simulink model "KTH_103002"  (Simulink 4.00)
settings: Solver=FixedStepDiscrete  StartTime=0.0  StopTime=5  RelTol=1e-3
values from neighbouring files (symbols this model uses):
  p2_1050 = [1.65 1.7 1.75 1.8 1.83 1.88 1.92 1.96 2.13 2.35 2.57 2.72 2.85 2.95]    [Comp1050_2.m]
  Pcomp_1050 = [690 790 880 1040 1160 1320 1580 1730 2970 5000 7960 9970 13200 16700]    [Comp1050_2.m]
  Qm_1050 = [2 2.5 3 4.5 5 6.5 8.5 10 20 35 55 65 85 100]    [Comp1050_2.m]
  T2_1050 = [99.2 103.5 107.2 110.7 111.8 112 111.7 100.4 116.5 131.5 136.4 147.4 149.6 155]    [Comp1050_2.m]
undefined symbols (not defined in the file or in its folder): conda, fan_cool, FC, fc_act, fc_blower_rec_H2, fc_blowera, fc_compressor, fc_condc, fc_coolstack, fc_current, fc_eqs, fc_evapcool, pump2, pump_cool, pump_re, radiator, vent
(part 1 of 2)
settings Model: LastModifiedBy=kharalds

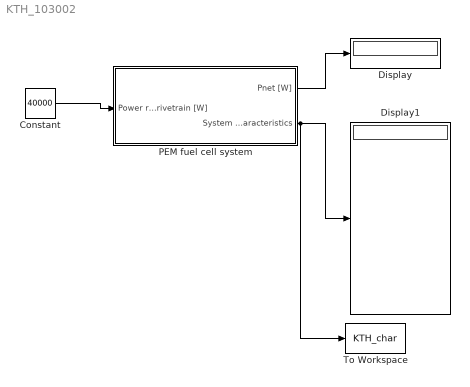
== system KTH_103002 ==
  Constant : Constant  Value=40000
  Display : Display
      settings: Format=short
  Display1 : Display
      settings: Format=short
  PEM fuel cell system : Subsystem
      settings: RTWFcnNameOpts=Auto  RTWFileNameOpts=Auto
  To Workspace : ToWorkspace  VariableName=KTH_char  SampleTime=-1  SaveFormat=Array
  wires:
  PEM fuel cell system/2(System characteristics) -> Display1/1, To Workspace/1
  PEM fuel cell system/1(Pnet [W]) -> Display/1
  Constant/1 -> PEM fuel cell system/1("Power request from drivetrain [W] ")

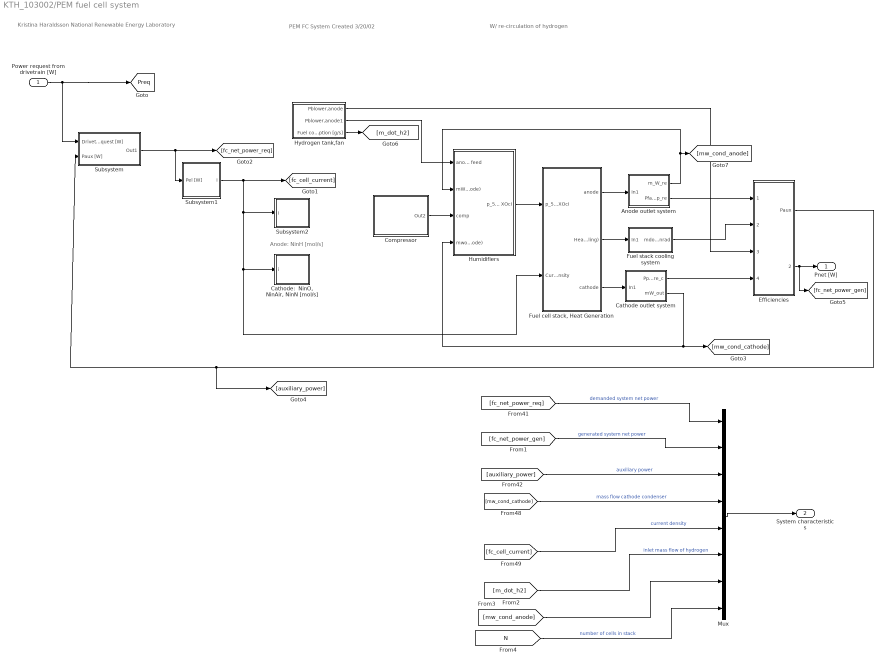
== system KTH_103002/PEM fuel cell system ==
  note: Kristina Haraldsson
      | National Renewable Energy Laboratory
  note: PEM FC System
      | Created  3/20/02
  note: W/ re-circulation of hydrogen
  note: Anode: NinH [mol/s]
  "Power request from drivetrain [W] " : Inport  Port=1  LatchInput=off
  Anode outlet system : Subsystem
      settings: RTWFcnNameOpts=Auto  RTWFileNameOpts=Auto
  Cathode outlet system : Subsystem
      settings: RTWFcnNameOpts=Auto  RTWFileNameOpts=Auto
  "Cathode:  NinO, NinAir, NinN [mol/s]" : Subsystem
      settings: RTWFcnNameOpts=Auto  RTWFileNameOpts=Auto
  "Compressor " : Subsystem
      settings: RTWFcnNameOpts=Auto  RTWFileNameOpts=Auto
  Efficiencies : Subsystem
      settings: RTWFcnNameOpts=Auto  RTWFileNameOpts=Auto
  "Fuel cell stack, Heat Generation" : Subsystem
      settings: RTWFcnNameOpts=Auto  RTWFileNameOpts=Auto
  Fuel stack cooling system : Subsystem
      settings: RTWFcnNameOpts=Auto  RTWFileNameOpts=Auto
  Humidifiers : Subsystem
      settings: RTWFcnNameOpts=Auto  RTWFileNameOpts=Auto
  Hydrogen tank,fan : Subsystem
      settings: RTWFcnNameOpts=Auto  RTWFileNameOpts=Auto
  Mux : Mux  Inputs=8
  Subsystem : Subsystem
      settings: RTWFcnNameOpts=Auto  RTWFileNameOpts=Auto
  Subsystem1 : Subsystem
      settings: RTWFcnNameOpts=Auto  RTWFileNameOpts=Auto
  Subsystem2 : Subsystem
      settings: RTWFcnNameOpts=Auto  RTWFileNameOpts=Auto
  Pnet [W] : Outport  Port=1
  System characteristics : Outport  Port=2
  tag scope: Preq=global
  wires:
  Humidifiers/1("p_56 anode feed p_57 cathode feed Psat Psatah Psatch XWaI,  XWcI  XOcI ") -> "Fuel cell stack, Heat Generation"/1("p_56, NinH, p_57, NinAir, Psat,Psatah,PsatchXWaI, XWcI, XOcI")
  "Compressor "/1(Out2) -> Humidifiers/3(comp)
  "Fuel cell stack, Heat Generation"/1(anode) -> Anode outlet system/1(In1)
  "Fuel cell stack, Heat Generation"/2(Heat_fc (fuel cell stack cooling)) -> Fuel stack cooling system/1(In1)
  Fuel stack cooling system/1(mdotW P_pump A Heat Qcool P_fanrad) -> Efficiencies/2(P_pump,cool P_fanrad)
  Anode outlet system/2(Pfan Ppump_re) -> Efficiencies/1("P_fan_,re, P_pump_re_a")
  Anode outlet system/1(m_W_re) -> Humidifiers/2(mW_out(anode)), [mw_cond_anode]
  "Fuel cell stack, Heat Generation"/3(cathode) -> Cathode outlet system/1(In1)
  Cathode outlet system/1(Ppump_re_c) -> Efficiencies/4(P_pump_re_c)
  Cathode outlet system/2(mW_out) -> Humidifiers/4(mwout(cathode)), [mw_cond_cathode]
  Hydrogen tank,fan/1(Pblower,anode) -> Efficiencies/3(P_fan,anode)
  Efficiencies/1(Paux) -> Subsystem/2(Paux [W]), [auxiliary_power]
  Subsystem/1(Out1) -> Subsystem1/1(Pel [W]), [fc_net_power_req]
  "Power request from drivetrain [W] "/1 -> Subsystem/1(Drivetrain Power Request [W]), [Preq]
  Subsystem1/1(i) -> Subsystem2/1(i), "Cathode:  NinO, NinAir, NinN [mol/s]"/1(i), "Fuel cell stack, Heat Generation"/2(Current density), [fc_cell_current]
  Efficiencies/2(Pnet [W]) -> Pnet [W]/1, [fc_net_power_gen]
  Hydrogen tank,fan/3(Fuel consumption [g/s]) -> [m_dot_h2]
  Hydrogen tank,fan/2(Pblower,anode1) -> Humidifiers/1(anode feed)
  [fc_net_power_req] -> Mux/1  "demanded system net power"
  [auxiliary_power] -> Mux/3  "auxiliary power"
  [mw_cond_cathode] -> Mux/4  "mass flow cathode condenser"
  [fc_cell_current] -> Mux/5  "current density"
  [fc_net_power_gen] -> Mux/2  "generated system net power"
  Mux/1 -> System characteristics/1
  [m_dot_h2] -> Mux/6  "inlet mass flow of hydrogen"
  [mw_cond_anode] -> Mux/7
  [N] -> Mux/8  "number of cells in stack"

== system KTH_103002/PEM fuel cell system/Anode outlet system ==
  note: FCSystem_H2/Anode outlet system
  In1 : Inport  Port=1  LatchInput=off
  Anode condenser : Subsystem
      settings: RTWFcnNameOpts=Auto  RTWFileNameOpts=Auto
  Mux : Mux  Inputs=2
  Mux1 : Mux  Inputs=2
  "Re-circulation: Blower_rec, pump" : Subsystem
      settings: RTWFcnNameOpts=Auto  RTWFileNameOpts=Auto
  Vent/Purge : Subsystem
      settings: RTWFcnNameOpts=Auto  RTWFileNameOpts=Auto
  m_W_re : Outport  Port=1
  Pfan Ppump_re : Outport  Port=2
  tag scope: NoutH=global
  wires:
  In1/1 -> Anode condenser/1(In1)
  Anode condenser/1(Out1) -> Vent/Purge/1(In1)
  Vent/Purge/1(Out1) -> "Re-circulation: Blower_rec, pump"/1(In1)
  "Re-circulation: Blower_rec, pump"/3(p_70) -> Mux/2
  "Re-circulation: Blower_rec, pump"/4(Pfan) -> Mux1/1
  "Re-circulation: Blower_rec, pump"/5(Ppump_re) -> Mux1/2
  Mux1/1 -> Pfan Ppump_re/1
  "Re-circulation: Blower_rec, pump"/1(m_W_re) -> m_W_re/1
  "Re-circulation: Blower_rec, pump"/2(NoutH_re) -> Mux/1
  Mux/1 -> [NoutH]

== system KTH_103002/PEM fuel cell system/Cathode outlet system ==
  note: FCSystem/Cathode outlet system
  In1 : Inport  Port=1  LatchInput=off
  Cathode condenser : Subsystem
      settings: RTWFcnNameOpts=Auto  RTWFileNameOpts=Auto
  Pump (cathode) : Subsystem
      settings: RTWFcnNameOpts=Auto  RTWFileNameOpts=Auto
  Ppump_re_c : Outport  Port=1
  mW_out : Outport  Port=2
  wires:
  In1/1 -> Cathode condenser/1(In1)
  Pump (cathode)/1(Ppump_re_c) -> Ppump_re_c/1
  Cathode condenser/1(mw_out1) -> Pump (cathode)/1(In1)
  Pump (cathode)/2(mW_out) -> mW_out/1

== system KTH_103002/PEM fuel cell system/Cathode:  NinO, NinAir, NinN [mol/s] ==
  note: Total cathode molar flow
  i : Inport  Port=1  LatchInput=off
  Constant : Constant  Value=FC.Lab.Stoich.vO
  Constant1 : Constant  Value=FC.Stack.Cell.Dim.A
  Constant2 : Constant  Value=FC.Stack.N
  Constant3 : Constant  Value=FC.Const.F
  Constant4 : Constant  Value=4
  Constant5 : Constant  Value=FC.Lab.Stoich.XON
  Constant6 : Constant  Value=FC.Lab.Stoich.XON
  Constant7 : Constant  Value=1
  Constant8 : Constant  Value=FC.Const.Mair
  Display{,1..3} (4 alike) : Display
      settings: Format=short
  Product : Product  Inputs=4  Multiplication=Element-wise(.*)  SaturateOnIntegerOverflow=on
  Product1 : Product  Inputs=*/  Multiplication=Element-wise(.*)  SaturateOnIntegerOverflow=on
  Product2 : Product  Inputs=2  Multiplication=Element-wise(.*)  SaturateOnIntegerOverflow=on
  Product3 : Product  Inputs=*/  Multiplication=Element-wise(.*)  SaturateOnIntegerOverflow=on
  Product4 : Product  Inputs=2  Multiplication=Element-wise(.*)  SaturateOnIntegerOverflow=on
  Product5 : Product  Inputs=2  Multiplication=Element-wise(.*)  SaturateOnIntegerOverflow=on
  Sum : Sum  Inputs=|+-  SaturateOnIntegerOverflow=on
  tag scope: NinAir=global, NinN=global, NinO=global
  wires:
  Constant1/1 -> Product/3
  Constant/1 -> Product/2
  i/1 -> Product/1
  Constant2/1 -> Product/4
  Product/1 -> Product1/1
  Constant4/1 -> Product2/2
  Product2/1 -> Product1/2
  Product1/1 -> Product3/1, [NinO], Display/1
  Constant5/1 -> Product3/2
  Product3/1 -> Product4/1, [NinAir], Display1/1, Product5/1
  Constant7/1 -> Sum/1
  Constant6/1 -> Sum/2
  Sum/1 -> Product4/2
  Product4/1 -> [NinN], Display2/1
  Constant3/1 -> Product2/1
  Constant8/1 -> Product5/2
  Product5/1 -> Display3/1

== system KTH_103002/PEM fuel cell system/Compressor  ==
  note: FCSystem_H2/Compressor
  "Initial value, 0.1 mole/s" : Memory  X0=0.1  InheritSampleTime=off
      settings: RTWStateStorageClass=Auto
  M_air [g/mol] : Constant  Value=FC.Const.Mair
  M_air [g/mol]1 : Constant  Value=FC.Lab.P.c
  Mass flow [g/s]  discharge pressure [bar(a)] CompOA1050 (Opcon) : Lookup  InputValues=[Qm_1050]  OutputValues=[p2_1050]
  Mass flow [g/s] Pcomp [W] CompOA1050 (Opcon) : Lookup  InputValues=[Qm_1050]  OutputValues=[Pcomp_1050]
  Mass flow [g/s] discharge temperature [C] CompOA1050 (Opcon)1 : Lookup  InputValues=[Qm_1050]  OutputValues=[T2_1050]
  Mux : Mux  Inputs=5
  P1 : Display
      settings: Format=short
  P2 : Display
      settings: Format=short
  Pcomp1 : Display
      settings: Format=short
  Product : Product  Inputs=2  Multiplication=Element-wise(.*)  SaturateOnIntegerOverflow=on
  Selector : Selector  InputType=Vector  ElementSrc=Internal  Elements=[4]  RowSrc=Internal  Rows=1  ColumnSrc=Internal  Columns=1  InputPortWidth=7
  fc_compressor.m : MATLABFcn  MATLABFcn=fc_compressor(u,FC.Lab.P.amb,FC.Lab.Temp.amb,FC.Const.eta1,FC.Const.etagen,FC.Lab.Stoich.RHo,FC.Lab.P.hum,FC.Lab.Temp.evap,FC.Lab.Temp.cell,FC.Stack.Pel)  OutputDimensions=7  OutputSignalType=auto  Output1D=on
  Out2 : Outport  Port=1
  tag scope: P_comp=global
  wires:
  M_air [g/mol]/1 -> Product/2
  Mux/1 -> fc_compressor.m/1
  Selector/1 -> Pcomp1/1, [P_comp]
  fc_compressor.m/1 -> Out2/1, Selector/1
  Mass flow [g/s]  discharge pressure [bar(a)] CompOA1050 (Opcon)/1 -> Mux/2, P2/1
  Mass flow [g/s] Pcomp [W] CompOA1050 (Opcon)/1 -> Mux/3
  [NinAir] -> "Initial value, 0.1 mole/s"/1
  "Initial value, 0.1 mole/s"/1 -> Mux/1, Product/1
  Product/1 -> Mass flow [g/s]  discharge pressure [bar(a)] CompOA1050 (Opcon)/1, Mass flow [g/s] Pcomp [W] CompOA1050 (Opcon)/1, Mass flow [g/s] discharge temperature [C] CompOA1050 (Opcon)1/1, P1/1
  Mass flow [g/s] discharge temperature [C] CompOA1050 (Opcon)1/1 -> Mux/4
  M_air [g/mol]1/1 -> Mux/5

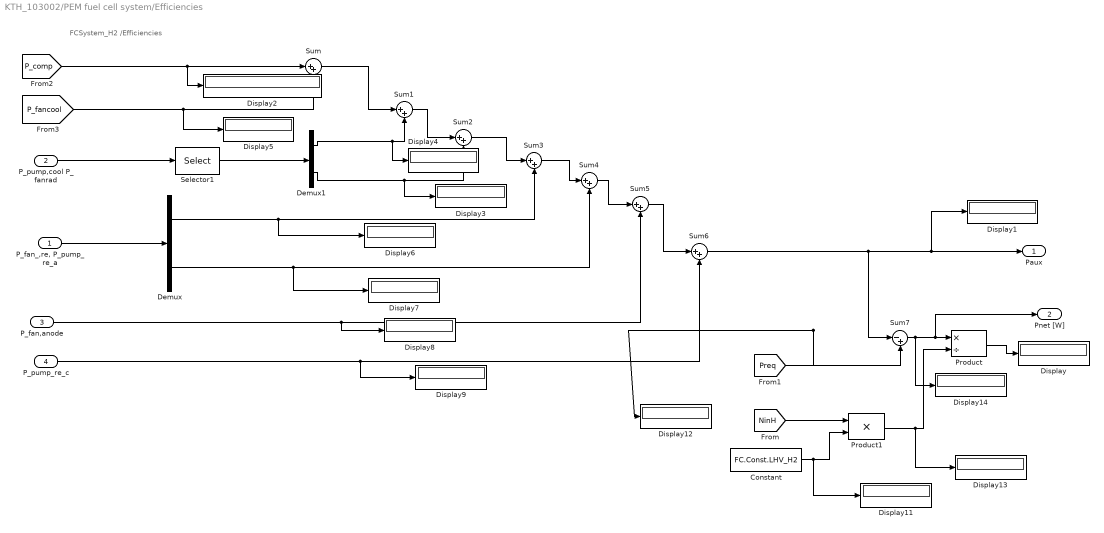
== system KTH_103002/PEM fuel cell system/Efficiencies ==
  note: FCSystem_H2
      | /Efficiencies
  "P_fan_,re, P_pump_re_a" : Inport  Port=1  LatchInput=off
  P_pump,cool P_fanrad : Inport  Port=2  LatchInput=off
  P_fan,anode : Inport  Port=3  LatchInput=off
  P_pump_re_c : Inport  Port=4  LatchInput=off
  Constant : Constant  Value=FC.Const.LHV_H2
  Demux : Demux  Outputs=2  BusSelectionMode=off
  Demux1 : Demux  Outputs=2  BusSelectionMode=off
  Display{,1..9,11..14} (14 alike) : Display
      Display settings: Format=short
      Display1 settings: Format=short
      Display11 settings: Format=short
      Display12 settings: Format=short
      Display13 settings: Format=short
      Display14 settings: Format=short
      Display3 settings: Format=short
      Display4 settings: Format=short
      Display5 settings: Format=short
      Display6 settings: Format=short
      Display7 settings: Format=short
      Display8 settings: Format=short
      Display9 settings: Format=short
  Product : Product  Inputs=*/  Multiplication=Element-wise(.*)  SaturateOnIntegerOverflow=on
  Product1 : Product  Inputs=2  Multiplication=Element-wise(.*)  SaturateOnIntegerOverflow=on
  Selector1 : Selector  InputType=Vector  ElementSrc=Internal  Elements=[2 6]  RowSrc=Internal  Rows=1  ColumnSrc=Internal  Columns=1  InputPortWidth=6
  Sum{,1..6} (7 alike) : Sum  Inputs=|++  SaturateOnIntegerOverflow=on
  Sum7 : Sum  Inputs=|-+  SaturateOnIntegerOverflow=on
  Paux : Outport  Port=1
  Pnet [W] : Outport  Port=2
  wires:
  P_pump,cool P_fanrad/1 -> Selector1/1
  [P_comp] -> Sum/1, Display2/1
  "P_fan_,re, P_pump_re_a"/1 -> Demux/1
  P_pump_re_c/1 -> Sum6/2, Display9/1
  P_fan,anode/1 -> Sum5/2, Display8/1
  Demux/1 -> Sum3/2, Display6/1
  Demux/2 -> Sum4/2, Display7/1
  [P_fancool] -> Sum/2, Display5/1
  Sum/1 -> Sum1/1
  Selector1/1 -> Demux1/1
  Demux1/1 -> Sum1/2, Display4/1
  Sum1/1 -> Sum2/1
  Demux1/2 -> Sum2/2, Display3/1
  Sum2/1 -> Sum3/1
  Sum3/1 -> Sum4/1
  Sum4/1 -> Sum5/1
  Sum5/1 -> Sum6/1
  Sum6/1 -> Sum7/1, Paux/1, Display1/1
  Sum7/1 -> Display14/1, Product/1, Pnet [W]/1
  [Preq] -> Sum7/2, Display12/1
  Constant/1 -> Product1/2, Display11/1
  [NinH] -> Product1/1
  Product1/1 -> Product/2, Display13/1
  Product/1 -> Display/1

== system KTH_103002/PEM fuel cell system/Fuel cell stack, Heat Generation ==
  note: FCSystem_H2
      | /Fuel cell stack, Heat generation
  note: NinWa NinHa NoutWag NoutHa
      | NinWc NinO NinN NoutWcg NWlgen
      | NoutWcl NoutO NoutN Nout_condc Nout_conda
  "p_56, NinH, p_57, NinAir, Psat,Psatah,PsatchXWaI, XWcI, XOcI" : Inport  Port=1  LatchInput=off
  Current density : Inport  Port=2  LatchInput=off
  Constant1 : Constant  Value=FC.Const.F
  Constant3 : Constant  Value=2
  Display{,1..3} (4 alike) : Display
      settings: Format=short
  Heat : Subsystem
      settings: RTWFcnNameOpts=Auto  RTWFileNameOpts=Auto
  J Water produced at cathode : Product  Inputs=/*  Multiplication=Element-wise(.*)  SaturateOnIntegerOverflow=on
  Mux1 : Mux  Inputs=5
  Product2 : Product  Inputs=2  Multiplication=Element-wise(.*)  SaturateOnIntegerOverflow=on
  fc_eqs : MATLABFcn  MATLABFcn=fc_eqs(u, FC.Stack.Cell.Dim.A, FC.Lab.P.a,FC.Lab.P.c,FC.Lab.P.amb,FC.Lab.Stoich.RHo,FC.Const.F,FC.Lab.Temp.cell,FC.Lab.Temp.ah,FC.Lab.Temp.ch,FC.Lab.Temp.amb,FC.Stack.Cell.Memb.Mm,FC.Stack.Cell.Memb.pdry,FC.Stack.Cell.Dim.tm,FC.Lab.Stoich.vO,FC.Lab.Stoich.vH,FC.Const.zw,FC.Stack.Pel,FC.Stack.N)  OutputDimensions=20  OutputSignalType=auto  Output1D=on
  flows : Selector  InputType=Vector  ElementSrc=Internal  Elements=[3 4 5 6 7 8 10 11 12 13 14 19 20]  RowSrc=Internal  Rows=1  ColumnSrc=Internal  Columns=1  InputPortWidth=20
  flows p_60 NoutWcg NoutWlgen NoutWcl NoutO NoutN Nout_condc : Selector  InputType=Vector  ElementSrc=Internal  Elements=[1 10 11 12 13 14 19]  RowSrc=Internal  Rows=1  ColumnSrc=Internal  Columns=1  InputPortWidth=20
  "p_61,NoutWag, NoutHa,NWAout,NoutWal" : Selector  InputType=Vector  ElementSrc=Internal  Elements=[2 5 6 16 17]  RowSrc=Internal  Rows=1  ColumnSrc=Internal  Columns=1  InputPortWidth=20
  anode : Outport  Port=1
  Heat_fc (fuel cell stack cooling) : Outport  Port=2
  cathode : Outport  Port=3
  tag scope: eta_fc=global
  wires:
  "p_56, NinH, p_57, NinAir, Psat,Psatah,PsatchXWaI, XWcI, XOcI"/1 -> Mux1/1
  "p_61,NoutWag, NoutHa,NWAout,NoutWal"/1 -> anode/1, Display/1
  Mux1/1 -> fc_eqs/1
  fc_eqs/1 -> "p_61,NoutWag, NoutHa,NWAout,NoutWal"/1, flows/1, flows p_60 NoutWcg NoutWlgen NoutWcl NoutO NoutN Nout_condc/1
  flows/1 -> Heat/1(In1 NinWa NinHa NoutWag NoutHa NinWc NinO NinN NoutWcg NoutWcl NoutO NoutN Nout_condc Nout_conda)
  Heat/1(Heat_fc) -> Heat_fc (fuel cell stack cooling)/1, Display3/1
  [NinO] -> Mux1/2
  [NinN] -> Mux1/3
  [lambda] -> Mux1/4
  Current density/1 -> Heat/2(Current density [A/cm2]), J Water produced at cathode/2
  Heat/2(eta_fc) -> [eta_fc], Display2/1
  flows p_60 NoutWcg NoutWlgen NoutWcl NoutO NoutN Nout_condc/1 -> cathode/1, Display1/1
  Constant1/1 -> Product2/1
  Constant3/1 -> Product2/2
  Product2/1 -> J Water produced at cathode/1
  J Water produced at cathode/1 -> Mux1/5

== system KTH_103002/PEM fuel cell system/Fuel stack cooling system ==
  note: FCSystem_H2
      | /Fuel stack cooling system
  note: Cooling medium: air
  note: Cooling medium: water
  In1 : Inport  Port=1  LatchInput=off
  Display : Display
      settings: Format=short
  Display1 : Display
      settings: Format=short
  Pump_cool : Subsystem
      settings: RTWFcnNameOpts=Auto  RTWFileNameOpts=Auto
  Radiator : Subsystem
      settings: RTWFcnNameOpts=Auto  RTWFileNameOpts=Auto
  fan_cool : Subsystem
      settings: RTWFcnNameOpts=Auto  RTWFileNameOpts=Auto
  fuel stack cooling mass flows : Subsystem
      settings: RTWFcnNameOpts=Auto  RTWFileNameOpts=Auto
  mdotW P_pump A Heat Qcool P_fanrad : Outport  Port=1
  tag scope: P_fancool=global
  wires:
  In1/1 -> fuel stack cooling mass flows/1(In1)
  fuel stack cooling mass flows/1(Cooling water flow [kg/s] Cooling air flow [kg/s]) -> Pump_cool/1(In1), fan_cool/1(m_A,T1,Q,etafc)
  fan_cool/1(P_fancool) -> Display/1, [P_fancool]
  Pump_cool/1(Out1) -> Radiator/1(In1)
  Radiator/1(Out2) -> mdotW P_pump A Heat Qcool P_fanrad/1, Display1/1

== system KTH_103002/PEM fuel cell system/Humidifiers ==
  note: FCSystem_H2/Humidifiers
  anode feed : Inport  Port=1  LatchInput=off
  mW_out(anode) : Inport  Port=2  LatchInput=off
  comp : Inport  Port=3  LatchInput=off
  mwout(cathode) : Inport  Port=4  LatchInput=off
  Constant : Constant  Value=FC.Lab.P.c
  Constant1 : Constant  Value=FC.Lab.P.a
  Evapcooler : Subsystem
      settings: RTWFcnNameOpts=Auto  RTWFileNameOpts=Auto
  Memory : Memory  X0=[0.00058799]  InheritSampleTime=off
      settings: RTWStateStorageClass=Auto
  Memory (former value  1.280458) : Memory  X0=0.04  InheritSampleTime=off
      settings: RTWStateStorageClass=Auto
  Mux : Mux  Inputs=6
  Selector : Selector  InputType=Vector  ElementSrc=Internal  Elements=[1 2 3 4 5 6 7 8 9 10 ]  RowSrc=Internal  Rows=1  ColumnSrc=Internal  Columns=1  InputPortWidth=25
  "p_56 anode feed p_57 cathode feed Psat Psatah Psatch XWaI,  XWcI  XOcI " : Outport  Port=1
  wires:
  anode feed/1 -> Evapcooler/1(anode feed Thyd p NinHa Pfan)
  Selector/1 -> "p_56 anode feed p_57 cathode feed Psat Psatah Psatch XWaI,  XWcI  XOcI "/1
  mW_out(anode)/1 -> Memory/1
  Memory/1 -> Evapcooler/2(mW_out(anode))
  mwout(cathode)/1 -> Memory (former value  1.280458)/1
  Evapcooler/1(Out1) -> Selector/1
  [psat_air] -> Mux/1
  [psatah] -> Mux/2
  [psatch] -> Mux/3
  [XWaI] -> Mux/4
  [XWcI] -> Mux/5
  [XOcI] -> Mux/6
  Mux/1 -> Evapcooler/7("Psat,Psatah, PsatchXWaI,  XWcI, XOcI")
  Memory (former value  1.280458)/1 -> Evapcooler/3(mW_out(cathode))
  Constant/1 -> Evapcooler/4(Pc)
  Constant1/1 -> Evapcooler/5(Pa)
  comp/1 -> Evapcooler/6(comp)

== system KTH_103002/PEM fuel cell system/Hydrogen tank,fan ==
  note: FCSystem_H2/Hydrogen tank, fan
  note: Fuel consumption
      | [mol/s]
  Constant : Constant  Value=FC.Const.MH
  Display : Display
      settings: Format=short
  Display1 : Display
      settings: Format=short
  Display2 : Display
      settings: Format=short
  Fcn : Fcn  Expr=u(4)
  Mux : Mux  Inputs=2
  NinH (initial fuel flow) [mol/s]  NinH (fuel cons.) [mol.s] : Selector  InputType=Vector  ElementSrc=Internal  Elements=[2]  RowSrc=Internal  Rows=1  ColumnSrc=Internal  Columns=1  InputPortWidth=2
  Product : Product  Inputs=2  Multiplication=Element-wise(.*)  SaturateOnIntegerOverflow=on
  Selector : Selector  InputType=Vector  ElementSrc=Internal  Elements=[1]  RowSrc=Internal  Rows=1  ColumnSrc=Internal  Columns=1  InputPortWidth=2
  Sum : Sum  Inputs=|+-  SaturateOnIntegerOverflow=on
  blowera.m : MATLABFcn  MATLABFcn=fc_blowera(u,FC.Const.etablow,FC.Stack.dpipe,FC.Stack.Lpipe,FC.Const.g,FC.Lab.P.blowa,FC.Lab.P.an,FC.Lab.P.a,FC.Lab.P.hum,FC.Lab.Temp.cell)  OutputDimensions=4  OutputSignalType=auto  Output1D=on
  Pblower,anode : Outport  Port=1
  Pblower,anode1 : Outport  Port=2
  Fuel consumption [g/s] : Outport  Port=3
  wires:
  blowera.m/1 -> Fcn/1, Pblower,anode1/1
  Fcn/1 -> Pblower,anode/1, Display2/1
  Mux/1 -> NinH (initial fuel flow) [mol/s]  NinH (fuel cons.) [mol.s]/1
  [NinH] -> Sum/1, blowera.m/1, Mux/1
  [NoutH] -> Selector/1
  Constant/1 -> Product/2
  NinH (initial fuel flow) [mol/s]  NinH (fuel cons.) [mol.s]/1 -> Product/1
  Product/1 -> Fuel consumption [g/s]/1
  Selector/1 -> Sum/2, Display/1
  Sum/1 -> Mux/2, Display1/1

== system KTH_103002/PEM fuel cell system/Subsystem ==
  note: Power Request
  Drivetrain Power Request [W] : Inport  Port=1  LatchInput=off
  Paux [W] : Inport  Port=2  LatchInput=off
  Display : Display
      settings: Format=short
  Display1 : Display
      settings: Format=short
  Display2 : Display
      settings: Format=short
  "Inverse of efficiency of DC/DC " : Constant  Orientation=up  Value=1/FC.Const.eta_DCDC
  Memory : Memory  X0=5000  InheritSampleTime=off
      settings: RTWStateStorageClass=Auto
  Preq=(Pel+Paux)/eta_DCDC : Product  Inputs=2  Multiplication=Element-wise(.*)  SaturateOnIntegerOverflow=on
  Sum1 : Sum  Inputs=|++  SaturateOnIntegerOverflow=on
  Out1 : Outport  Port=1
  wires:
  Drivetrain Power Request [W]/1 -> Display2/1, Sum1/1
  Sum1/1 -> Preq=(Pel+Paux)/eta_DCDC/1, Display/1
  "Inverse of efficiency of DC/DC "/1 -> Preq=(Pel+Paux)/eta_DCDC/2
  Preq=(Pel+Paux)/eta_DCDC/1 -> Display1/1, Out1/1
  Paux [W]/1 -> Memory/1
  Memory/1 -> Sum1/2

== system KTH_103002/PEM fuel cell system/Subsystem1 ==
  Pel [W] : Inport  Port=1  LatchInput=off
  Anode init : Subsystem
      settings: RTWFcnNameOpts=Auto  RTWFileNameOpts=Auto
  Cathode Overpotential : Subsystem
      settings: RTWFcnNameOpts=Auto  RTWFileNameOpts=Auto
  Cathode oxygen molar fraction : Subsystem
      settings: RTWFcnNameOpts=Auto  RTWFileNameOpts=Auto
  Cathode water molar fraction : Subsystem
      settings: RTWFcnNameOpts=Auto  RTWFileNameOpts=Auto
  Constant : Constant  Value=FC.Stack.N
  Demux : Demux  Outputs=3  BusSelectionMode=off
  Display{1..4} (4 alike) : Display
      settings: Format=short
  Membrane conductivity : Subsystem
      settings: RTWFcnNameOpts=Auto  RTWFileNameOpts=Auto
  Membrane resistance : Subsystem
      settings: RTWFcnNameOpts=Auto  RTWFileNameOpts=Auto
  Mux : Mux  Inputs=4
  Saturation pressure  cathode humidifier : Subsystem
      settings: RTWFcnNameOpts=Auto  RTWFileNameOpts=Auto
  fc_current : MATLABFcn  MATLABFcn=fc_current(u,FC.Lab.P.c,FC.Lab.P.a,FC.Stack.Cell.Dim.tm,FC.Const.F,FC.Const.jo,FC.Const.Voc,FC.Const.R2,FC.Stack.Cell.Dim.A,FC.Lab.Temp.cell,FC.Lab.Temp.ah,FC.Lab.Temp.ch)  OutputDimensions=3  OutputSignalType=auto  Output1D=on
  i : Outport  Port=1
  tag scope: Ecell=global, N=global, Po=global, Rm=global
  wires:
  Membrane conductivity/1(Sigma) -> Membrane resistance/1(sigma)
  Anode init/1(lambda) -> Membrane conductivity/1(lambda)
  Membrane resistance/1(Rm [ohm/cm2]) -> [Rm], Mux/1
  Saturation pressure  cathode humidifier/1(psatch) -> Cathode water molar fraction/1(psatch [bar])
  Cathode water molar fraction/1(XWcI [-]) -> Cathode Overpotential/2(XWcI), Cathode oxygen molar fraction/1(XWcI [-]1)
  Cathode oxygen molar fraction/1(XOcI [-]) -> Cathode Overpotential/1(XOcI)
  Cathode Overpotential/1(Po) -> [Po], Mux/2
  Mux/1 -> fc_current/1
  Pel [W]/1 -> Mux/3
  fc_current/1 -> Demux/1
  Demux/2 -> [Ecell], Display1/1
  Demux/1 -> i/1, Display4/1
  Demux/3 -> [N], Display2/1
  Constant/1 -> Mux/4, Display3/1

== system KTH_103002/PEM fuel cell system/Subsystem2 ==
  note: Total anode molar flow
  i : Inport  Port=1  LatchInput=off
  Constant : Constant  Value=FC.Lab.Stoich.vH
  Constant1 : Constant  Value=FC.Stack.Cell.Dim.A
  Constant2 : Constant  Value=FC.Stack.N
  Constant3 : Constant  Value=FC.Const.F
  Constant4 : Constant  Value=2
  Constant5 : Constant  Value=FC.Const.MH
  Display : Display
      settings: Format=short
  Display1 : Display
      settings: Format=short
  Product : Product  Inputs=4  Multiplication=Element-wise(.*)  SaturateOnIntegerOverflow=on
  Product1 : Product  Inputs=*/  Multiplication=Element-wise(.*)  SaturateOnIntegerOverflow=on
  Product2 : Product  Inputs=2  Multiplication=Element-wise(.*)  SaturateOnIntegerOverflow=on
  Product3 : Product  Inputs=2  Multiplication=Element-wise(.*)  SaturateOnIntegerOverflow=on
  tag scope: NinH=global
  wires:
  Constant1/1 -> Product/3
  Constant/1 -> Product/2
  i/1 -> Product/1
  Constant2/1 -> Product/4
  Product/1 -> Product1/1
  Constant3/1 -> Product2/1
  Constant4/1 -> Product2/2
  Product2/1 -> Product1/2
  Product1/1 -> [NinH], Display/1, Product3/1
  Constant5/1 -> Product3/2
  Product3/1 -> Display1/1

== system KTH_103002/PEM fuel cell system/Anode outlet system/Anode condenser ==
  note: FCSystem_H2/Anode outlet system/Anode condenser
  In1 : Inport  Port=1  LatchInput=off
  conda : MATLABFcn  MATLABFcn=conda(u,FC.Const.ex,FC.Lab.Temp.amb,FC.Lab.Temp.cond,FC.Lab.Temp.cell)  OutputDimensions=6  OutputSignalType=auto  Output1D=on
  Out1 : Outport  Port=1
  wires:
  In1/1 -> conda/1
  conda/1 -> Out1/1

== system KTH_103002/PEM fuel cell system/Anode outlet system/Re-circulation: Blower_rec, pump ==
  note: FCSystem_H2/Anode outlet system/Blower, pump
  In1 : Inport  Port=1  LatchInput=off
  Demux : Demux  Outputs=2  BusSelectionMode=off
  Demux1 : Demux  Outputs=3  BusSelectionMode=off
  Memory : Memory  X0=0.06848  InheritSampleTime=off
      settings: RTWStateStorageClass=Auto
  Memory1 : Memory  X0=2.59  InheritSampleTime=off
      settings: RTWStateStorageClass=Auto
  Selector1 : Selector  InputType=Vector  ElementSrc=Internal  Elements=[2 3 4]  RowSrc=Internal  Rows=1  ColumnSrc=Internal  Columns=1  InputPortWidth=5
  Selector2 : Selector  InputType=Vector  ElementSrc=Internal  Elements=[1 2]  RowSrc=Internal  Rows=1  ColumnSrc=Internal  Columns=1  InputPortWidth=5
  fc_blower_rec_H2 re-circulation of hydrogen : MATLABFcn  MATLABFcn=fc_blower_rec_H2(u,FC.Const.etablow,FC.Lab.Temp.cell,FC.Stack.dpipe,FC.Stack.Lpipe,FC.Lab.P.blowr,FC.Const.g,FC.Const.MH)  OutputDimensions=5  OutputSignalType=auto  Output1D=on
  pump_re (re-circulation of water from the anode) : MATLABFcn  MATLABFcn=pump_re(u,FC.Lab.Temp.cond,FC.Const.g,FC.Stack.dpipe,FC.Stack.Lpipe,FC.Const.etapump)  OutputDimensions=5  OutputSignalType=auto  Output1D=on
  m_W_re : Outport  Port=1
  NoutH_re : Outport  Port=2
  p_70 : Outport  Port=3
  Pfan : Outport  Port=4
  Ppump_re : Outport  Port=5
  wires:
  In1/1 -> pump_re (re-circulation of water from the anode)/1, fc_blower_rec_H2 re-circulation of hydrogen/1
  pump_re (re-circulation of water from the anode)/1 -> Selector2/1
  Selector2/1 -> Demux/1
  Demux/1 -> Ppump_re/1
  Demux/2 -> m_W_re/1
  Selector1/1 -> Demux1/1
  Demux1/2 -> Memory1/1
  fc_blower_rec_H2 re-circulation of hydrogen/1 -> Selector1/1
  Demux1/1 -> Memory/1
  Memory/1 -> NoutH_re/1
  Memory1/1 -> p_70/1
  Demux1/3 -> Pfan/1

== system KTH_103002/PEM fuel cell system/Anode outlet system/Vent/Purge ==
  note: FCSystem_H2/Anode outlet system/Purge
  In1 : Inport  Port=1  LatchInput=off
  vent : MATLABFcn  MATLABFcn=vent(u,FC.Const.ex)  OutputDimensions=10  OutputSignalType=auto  Output1D=on
  Out1 : Outport  Port=1
  wires:
  In1/1 -> vent/1
  vent/1 -> Out1/1

== system KTH_103002/PEM fuel cell system/Cathode outlet system/Cathode condenser ==
  note: FCSystem/Cathode outlet system/Cathode condenser
  In1 : Inport  Port=1  LatchInput=off
  Mux : Mux  Inputs=2
  Saturation temperature : Subsystem
      settings: RTWFcnNameOpts=Auto  RTWFileNameOpts=Auto
  Selector : Selector  InputType=Vector  ElementSrc=Internal  Elements=[1]  RowSrc=Internal  Rows=1  ColumnSrc=Internal  Columns=1  InputPortWidth=7
  To Workspace : ToWorkspace  VariableName=condc  SampleTime=-1  SaveFormat=Array
  fc_condc : MATLABFcn  MATLABFcn=fc_condc(u,FC.Lab.Temp.amb,FC.Lab.Temp.cond,FC.Lab.Temp.ch,FC.Lab.Temp.cell)  OutputDimensions=7  OutputSignalType=auto  Output1D=on
  mw_out : Selector  InputType=Vector  ElementSrc=Internal  Elements=[4]  RowSrc=Internal  Rows=1  ColumnSrc=Internal  Columns=1  InputPortWidth=7
  mw_out1 : Outport  Port=1
  wires:
  In1/1 -> Mux/1, Selector/1
  fc_condc/1 -> mw_out/1, To Workspace/1
  mw_out/1 -> mw_out1/1
  Mux/1 -> fc_condc/1
  Saturation temperature/1(Temp [K]) -> Mux/2
  Selector/1 -> Saturation temperature/1(pressure [bar])

== system KTH_103002/PEM fuel cell system/Cathode outlet system/Pump (cathode) ==
  note: FCSystem/Cathode outlet system/Pump (cathode)
  note: mw_out
      | condensed water from
      |  the cathode
  In1 : Inport  Port=1  LatchInput=off
  Selector : Selector  InputType=Vector  ElementSrc=Internal  Elements=[2]  RowSrc=Internal  Rows=1  ColumnSrc=Internal  Columns=1  InputPortWidth=2
  Selector1 : Selector  InputType=Vector  ElementSrc=Internal  Elements=[1]  RowSrc=Internal  Rows=1  ColumnSrc=Internal  Columns=1  InputPortWidth=2
  To Workspace : ToWorkspace  VariableName=pump_re_c  SampleTime=-1  SaveFormat=Array
  pump2 (re-circulation of water from the cathode) : MATLABFcn  MATLABFcn=pump2(u,FC.Lab.Temp.cond,FC.Const.g,FC.Stack.dpipe,FC.Stack.Lpipe,FC.Const.etapump)  OutputDimensions=2  OutputSignalType=auto  Output1D=on
  Ppump_re_c : Outport  Port=1
  mW_out : Outport  Port=2
  wires:
  In1/1 -> pump2 (re-circulation of water from the cathode)/1
  pump2 (re-circulation of water from the cathode)/1 -> To Workspace/1, Selector/1, Selector1/1
  Selector/1 -> Ppump_re_c/1
  Selector1/1 -> mW_out/1

== system KTH_103002/PEM fuel cell system/Fuel cell stack, Heat Generation/Heat ==
  note: Heat & efficiency of fuel cell stack
  In1 NinWa NinHa NoutWag NoutHa NinWc NinO NinN NoutWcg NoutWcl NoutO NoutN Nout_condc Nout_conda : Inport  Port=1  LatchInput=off
  Current density [A/cm2] : Inport  Port=2  LatchInput=off
  Demux : Demux  Outputs=13  BusSelectionMode=off
  Fuel cell efficiency : Subsystem
      settings: RTWFcnNameOpts=Auto  RTWFileNameOpts=Auto
  Heat generation [W] : Subsystem
      settings: RTWFcnNameOpts=Auto  RTWFileNameOpts=Auto
  Latent heat [W] : Subsystem
      settings: RTWFcnNameOpts=Auto  RTWFileNameOpts=Auto
  Reaction heat [W] : Subsystem
      settings: RTWFcnNameOpts=Auto  RTWFileNameOpts=Auto
  Sensible heat [W] : Subsystem
      settings: RTWFcnNameOpts=Auto  RTWFileNameOpts=Auto
  Sum : Sum  Inputs=|++  SaturateOnIntegerOverflow=on
  Heat_fc : Outport  Port=1
  eta_fc : Outport  Port=2
  wires:
  In1 NinWa NinHa NoutWag NoutHa NinWc NinO NinN NoutWcg NoutWcl NoutO NoutN Nout_condc Nout_conda/1 -> Demux/1
  Demux/1 -> Sensible heat [W]/1(NinWa)
  Demux/2 -> Sensible heat [W]/2(NinHa)
  Demux/3 -> Sensible heat [W]/3(NoutWag)
  Demux/4 -> Sensible heat [W]/4(NoutHa)
  Demux/5 -> Sensible heat [W]/5(NinWc)
  Demux/6 -> Sensible heat [W]/6(NinO)
  Demux/7 -> Sensible heat [W]/7(NInN)
  Demux/8 -> Sensible heat [W]/8(NoutWcg)
  Demux/9 -> Sensible heat [W]/9(NoutWcl)
  Demux/10 -> Sensible heat [W]/10(NoutO)
  Demux/11 -> Sensible heat [W]/11(NoutN)
  Demux/12 -> Sum/1
  Demux/13 -> Sum/2
  Sum/1 -> Latent heat [W]/1(NWcond)
  Current density [A/cm2]/1 -> Reaction heat [W]/1(Current density)
  [Ecell] -> Reaction heat [W]/2(Ecell), Fuel cell efficiency/2(Ecell)
  Sensible heat [W]/1(sensin) -> Heat generation [W]/1(sensin)
  Sensible heat [W]/2(sensout) -> Heat generation [W]/2(sensout)
  Latent heat [W]/1(latheat [W]) -> Heat generation [W]/3(latheat)
  Reaction heat [W]/1(reaheat [W]) -> Heat generation [W]/4(reaheat)
  Heat generation [W]/1(Heat_fc) -> Heat_fc/1
  Reaction heat [W]/2(Hr [J/mol]) -> Fuel cell efficiency/1(Hr)
  Fuel cell efficiency/1(eta_fc) -> eta_fc/1

== system KTH_103002/PEM fuel cell system/Fuel stack cooling system/Pump_cool ==
  note: FCSystem_H2/fuel stack cooling system/Pumpcool
  In1 : Inport  Port=1  LatchInput=off
  pump_cool.m : MATLABFcn  MATLABFcn=pump_cool(u,FC.Lab.Temp.cool,FC.Const.g,FC.Stack.dpipefc,FC.Stack.Lpipefc,FC.Const.etapump,FC.Lab.Temp.cell,FC.Stack.Lpipe,FC.Stack.dpipe,FC.Stack.N)  OutputDimensions=6  OutputSignalType=auto  Output1D=on
  Out1 : Outport  Port=1
  wires:
  In1/1 -> pump_cool.m/1
  pump_cool.m/1 -> Out1/1

== system KTH_103002/PEM fuel cell system/Fuel stack cooling system/Radiator ==
  note: FCSystem_H2/Cooling system/Radiator
  In1 : Inport  Port=1  LatchInput=off
  radiator.m : MATLABFcn  MATLABFcn=radiator(u,FC.Lab.Temp.amb,FC.Lab.Temp.rad,FC.Const.U,FC.Lab.Temp.cool,FC.Const.kw,FC.Stack.dpipe,FC.Stack.Lpipe,FC.Const.etablow,FC.Lab.Temp.cell,FC.Const.g,FC.Stack.drad,FC.Stack.Lrad,FC.Const.Nrad)  OutputDimensions=6  OutputSignalType=auto  Output1D=on
  Out2 : Outport  Port=1
  wires:
  radiator.m/1 -> Out2/1
  In1/1 -> radiator.m/1

== system KTH_103002/PEM fuel cell system/Fuel stack cooling system/fan_cool ==
  note: FCSystem_H2/Cooling system/Fan_cool
  m_A,T1,Q,etafc : Inport  Port=1  LatchInput=off
  Selector : Selector  InputType=Vector  ElementSrc=Internal  Elements=[2]  RowSrc=Internal  Rows=1  ColumnSrc=Internal  Columns=1  InputPortWidth=4
  fan_cool.m : MATLABFcn  MATLABFcn=fan_cool(u,FC.Lab.Temp.cool,FC.Lab.Temp.cell,FC.Const.g,FC.Stack.dpipefc,FC.Stack.Lpipefc,FC.Const.etablow,FC.Lab.P.amb,FC.Lab.P.blowr)  OutputDimensions=4  OutputSignalType=auto  Output1D=on
  P_fancool : Outport  Port=1
  wires:
  m_A,T1,Q,etafc/1 -> fan_cool.m/1
  fan_cool.m/1 -> Selector/1
  Selector/1 -> P_fancool/1

== system KTH_103002/PEM fuel cell system/Fuel stack cooling system/fuel stack cooling mass flows ==
  note: FCSystem_H2/Fuel stack cooling system/Fuel stack cooling, mass flows
  In1 : Inport  Port=1  LatchInput=off
  fc_coolstack.m : MATLABFcn  MATLABFcn=fc_coolstack(u,FC.Lab.Temp.cool,FC.Lab.Temp.amb,FC.Lab.Temp.cell)  OutputDimensions=4  OutputSignalType=auto  Output1D=on
  Cooling water flow [kg/s] Cooling air flow [kg/s] : Outport  Port=1
  wires:
  In1/1 -> fc_coolstack.m/1
  fc_coolstack.m/1 -> Cooling water flow [kg/s] Cooling air flow [kg/s]/1

== system KTH_103002/PEM fuel cell system/Humidifiers/Evapcooler ==
  note: FCSystem_H2/Humidifiers/evapcooler
  anode feed Thyd p NinHa Pfan : Inport  Port=1  LatchInput=off
  mW_out(anode) : Inport  Port=2  LatchInput=off
  mW_out(cathode) : Inport  Port=3  LatchInput=off
  Pc : Inport  Port=4  LatchInput=off
  Pa : Inport  Port=5  LatchInput=off
  comp : Inport  Port=6  LatchInput=off
  "Psat,Psatah, PsatchXWaI,  XWcI, XOcI" : Inport  Port=7  LatchInput=off
  Ambient air : Subsystem
      settings: RTWFcnNameOpts=Auto  RTWFileNameOpts=Auto
  Mux1 : Mux  Inputs=7
  Selector : Selector  InputType=Vector  ElementSrc=Internal  Elements=[1 2 3]  RowSrc=Internal  Rows=1  ColumnSrc=Internal  Columns=1  InputPortWidth=4
  fc_evapcool : MATLABFcn  MATLABFcn=fc_evapcool(u,FC.Lab.Temp.cell,FC.Lab.Temp.evap,FC.Lab.P.hum,FC.Lab.Temp.hyd,FC.Lab.Stoich.RHah,FC.Lab.Stoich.RHch,FC.Lab.P.an,FC.Lab.Temp.cond)  OutputDimensions=25  OutputSignalType=auto  Output1D=on
  Out1 : Outport  Port=1
  wires:
  mW_out(anode)/1 -> Mux1/2
  Pa/1 -> Mux1/5
  Pc/1 -> Mux1/4
  mW_out(cathode)/1 -> Mux1/3
  Mux1/1 -> fc_evapcool/1
  fc_evapcool/1 -> Out1/1
  anode feed Thyd p NinHa Pfan/1 -> Selector/1
  Selector/1 -> Mux1/1
  comp/1 -> Mux1/6
  "Psat,Psatah, PsatchXWaI,  XWcI, XOcI"/1 -> Mux1/7

== system KTH_103002/PEM fuel cell system/Subsystem1/Anode init ==
  note: Anode
      | Saturation pressure, water fraction, activity, lambda
  Anode water molar fraction : Subsystem
      settings: RTWFcnNameOpts=Auto  RTWFileNameOpts=Auto
  Saturation pressure  anode humidifier : Subsystem
      settings: RTWFcnNameOpts=Auto  RTWFileNameOpts=Auto
  Subsystem2 : Subsystem
      settings: RTWFcnNameOpts=Auto  RTWFileNameOpts=Auto
  fc_act.m : MATLABFcn  MATLABFcn=fc_act(u)  OutputDimensions=1  OutputSignalType=auto  Output1D=on
  lambda : Outport  Port=1
  tag scope: lambda=global
  wires:
  Saturation pressure  anode humidifier/1(psatah) -> Anode water molar fraction/1(psatah [bar]), Subsystem2/2(psatah [bar])
  Anode water molar fraction/1(XWaI [-]) -> Subsystem2/1(XWaI [-])
  Subsystem2/1(a) -> fc_act.m/1
  fc_act.m/1 -> lambda/1, [lambda]

== system KTH_103002/PEM fuel cell system/Subsystem1/Cathode Overpotential ==
  note: Cathode overpotential
  XOcI : Inport  Port=1  LatchInput=off
  XWcI : Inport  Port=2  LatchInput=off
  Constant : Constant  Value=FC.Lab.P.c
  Constant1 : Constant  Value=1
  Product : Product  Inputs=*/  Multiplication=Element-wise(.*)  SaturateOnIntegerOverflow=on
  Product1 : Product  Inputs=2  Multiplication=Element-wise(.*)  SaturateOnIntegerOverflow=on
  Sum : Sum  Inputs=|+-  SaturateOnIntegerOverflow=on
  Po : Outport  Port=1
  wires:
  Constant1/1 -> Sum/1
  XWcI/1 -> Sum/2
  XOcI/1 -> Product/1
  Sum/1 -> Product/2
  Product/1 -> Product1/1
  Constant/1 -> Product1/2
  Product1/1 -> Po/1

== system KTH_103002/PEM fuel cell system/Subsystem1/Cathode oxygen molar fraction ==
  note: Oxygen molar fraction in the cathode inlet stream
  XWcI [-]1 : Inport  Port=1  LatchInput=off
  0.21 : Constant  Value=FC.Lab.Stoich.XON
  Constant1 : Constant  Value=1
  Product2 : Product  Inputs=2  Multiplication=Element-wise(.*)  SaturateOnIntegerOverflow=on
  Sum : Sum  Inputs=|+-  SaturateOnIntegerOverflow=on
  XOcI [-] : Outport  Port=1
  tag scope: XOcI=global
  wires:
  Product2/1 -> XOcI [-]/1, [XOcI]
  Constant1/1 -> Sum/1
  XWcI [-]1/1 -> Sum/2
  Sum/1 -> Product2/1
  0.21/1 -> Product2/2

== system KTH_103002/PEM fuel cell system/Subsystem1/Cathode water molar fraction ==
  note: Water molar fraction in the cathode inlet stream
  psatch [bar] : Inport  Port=1  LatchInput=off
  Constant1 : Constant  Value=FC.Lab.P.c
  Constant3 : Constant  Value=FC.Lab.Stoich.RHch
  Constant4 : Constant  Value=100
  Product : Product  Inputs=*/  Multiplication=Element-wise(.*)  SaturateOnIntegerOverflow=on
  Product1 : Product  Inputs=*/  Multiplication=Element-wise(.*)  SaturateOnIntegerOverflow=on
  Product2 : Product  Inputs=2  Multiplication=Element-wise(.*)  SaturateOnIntegerOverflow=on
  XWcI [-] : Outport  Port=1
  tag scope: XWcI=global
  wires:
  Constant3/1 -> Product1/1
  Constant4/1 -> Product1/2
  psatch [bar]/1 -> Product/1
  Constant1/1 -> Product/2
  Product1/1 -> Product2/1
  Product/1 -> Product2/2
  Product2/1 -> XWcI [-]/1, [XWcI]

== system KTH_103002/PEM fuel cell system/Subsystem1/Membrane conductivity ==
  note: Membrane conductivity
      | Nafion 117
  lambda : Inport  Port=1  LatchInput=off
  Constant : Constant  Value=0.005139
  Constant1 : Constant  Value=0.00326
  Constant2 : Constant  Value=303
  Constant3 : Constant  Value=273
  Constant4 : Constant  Value=1268
  Constant5 : Constant  Value=FC.Lab.Temp.cell
  Constant6 : Constant  Value=1
  Constant8 : Constant  Value=1
  Math Function : Math  Operator=exp  OutputSignalType=auto
  Product : Product  Inputs=2  Multiplication=Element-wise(.*)  SaturateOnIntegerOverflow=on
  Product1 : Product  Inputs=2  Multiplication=Element-wise(.*)  SaturateOnIntegerOverflow=on
  Product2 : Product  Inputs=*/  Multiplication=Element-wise(.*)  SaturateOnIntegerOverflow=on
  Product3 : Product  Inputs=*/  Multiplication=Element-wise(.*)  SaturateOnIntegerOverflow=on
  Product4 : Product  Inputs=2  Multiplication=Element-wise(.*)  SaturateOnIntegerOverflow=on
  Sum : Sum  Inputs=|+-  SaturateOnIntegerOverflow=on
  Sum1 : Sum  Inputs=|++  SaturateOnIntegerOverflow=on
  Sum2 : Sum  Inputs=|+-  SaturateOnIntegerOverflow=on
  Sigma : Outport  Port=1
  wires:
  lambda/1 -> Product/1
  Constant/1 -> Product/2
  Product/1 -> Sum/1
  Constant1/1 -> Sum/2
  Sum/1 -> Product1/1
  Constant6/1 -> Product2/1
  Constant2/1 -> Product2/2
  Constant8/1 -> Product3/1
  Sum1/1 -> Product3/2
  Constant3/1 -> Sum1/1
  Constant5/1 -> Sum1/2
  Product2/1 -> Sum2/1
  Product3/1 -> Sum2/2
  Constant4/1 -> Product4/1
  Sum2/1 -> Product4/2
  Product4/1 -> Math Function/1
  Math Function/1 -> Product1/2
  Product1/1 -> Sigma/1

== system KTH_103002/PEM fuel cell system/Subsystem1/Membrane resistance ==
  note: Membrane resistance [ohm/cm2]
  sigma : Inport  Port=1  LatchInput=off
  Constant : Constant  Value=FC.Stack.Cell.Dim.tm
  Product : Product  Inputs=*/  Multiplication=Element-wise(.*)  SaturateOnIntegerOverflow=on
  Rm [ohm/cm2] : Outport  Port=1
  wires:
  Constant/1 -> Product/1
  sigma/1 -> Product/2
  Product/1 -> Rm [ohm/cm2]/1

== system KTH_103002/PEM fuel cell system/Subsystem1/Saturation pressure  cathode humidifier ==
  note: Saturation pressure of water in the cathode humidifier
      | NOTE: [bar]
      | Data from "Anlaggnings- och apparatteknik", Westerlund, T., Abo Akademi, Finland, 1998
  Cathode humidifier temperature [C] : Constant  Value=FC.Lab.Temp.ch
  Cathode humidifier temperature [C]1 : Constant  Value=FC.Lab.Temp.ch
  Constant : Constant  Value=11.78
  Constant1 : Constant  Value=99.64
  Constant2 : Constant  Value=230
  Math Function : Math  Operator=exp  OutputSignalType=auto
  Product : Product  Inputs=*/  Multiplication=Element-wise(.*)  SaturateOnIntegerOverflow=on
  Product1 : Product  Inputs=2  Multiplication=Element-wise(.*)  SaturateOnIntegerOverflow=on
  Sum : Sum  Inputs=|+-  SaturateOnIntegerOverflow=on
  Sum1 : Sum  Inputs=|++  SaturateOnIntegerOverflow=on
  psatch : Outport  Port=1
  tag scope: psatch=global
  wires:
  Cathode humidifier temperature [C]/1 -> Sum/1
  Constant1/1 -> Sum/2
  Cathode humidifier temperature [C]1/1 -> Sum1/1
  Constant2/1 -> Sum1/2
  Sum/1 -> Product/1
  Sum1/1 -> Product/2
  Constant/1 -> Product1/2
  Product/1 -> Product1/1
  Product1/1 -> Math Function/1
  Math Function/1 -> psatch/1, [psatch]

== system KTH_103002/PEM fuel cell system/Cathode outlet system/Cathode condenser/Saturation temperature ==
  note: Saturation temperature [K]
      | --------------------------------------------
      |  Data from L. Wester, 1998
      |  valid: 273.16<=Tsat<600 K and 0.000611<=p<12.33 MPa
      |
      | A=42.6776;
      | B=-3892.70;
      | C=-9.48654;
      |
      | T=A+B/(log(p)+C);
  pressure [bar] : Inport  Port=1  LatchInput=off
  A : Constant  Value=42.6776
  B : Constant  Value=-3892.70
  C : Constant  Value=-9.48654
  Constant : Constant  Value=100000
  Math Function : Math  Operator=log  OutputSignalType=auto
  Product : Product  Inputs=*/  Multiplication=Element-wise(.*)  SaturateOnIntegerOverflow=on
  Sum : Sum  Inputs=|++  SaturateOnIntegerOverflow=on
  Sum1 : Sum  Inputs=|++  SaturateOnIntegerOverflow=on
  "[bar] to [MPa]" : Product  Inputs=*/  Multiplication=Element-wise(.*)  SaturateOnIntegerOverflow=on
  Temp [K] : Outport  Port=1
  wires:
  pressure [bar]/1 -> "[bar] to [MPa]"/1
  Constant/1 -> "[bar] to [MPa]"/2
  A/1 -> Sum/1
  B/1 -> Product/1
  C/1 -> Sum1/2
  Sum1/1 -> Temp [K]/1
  Product/1 -> Sum/2
  Sum/1 -> Sum1/1
  "[bar] to [MPa]"/1 -> Math Function/1
  Math Function/1 -> Product/2

== system KTH_103002/PEM fuel cell system/Fuel cell stack, Heat Generation/Heat/Fuel cell efficiency ==
  note: Fuel cell efficiency
      | -----------------------------
      | eta_fc=(-2*F*Ecell)/Hr;
  Hr : Inport  Port=1  LatchInput=off
  Ecell : Inport  Port=2  LatchInput=off
  Constant : Constant  Value=FC.Const.F
  Constant1 : Constant  Value=2
  Gain : Gain  Gain=-1  Multiplication=Element-wise(K.*u)  SaturateOnIntegerOverflow=on
  Product : Product  Inputs=/*  Multiplication=Element-wise(.*)  SaturateOnIntegerOverflow=on
  Product2 : Product  Inputs=3  Multiplication=Element-wise(.*)  SaturateOnIntegerOverflow=on
  eta_fc : Outport  Port=1
  wires:
  Ecell/1 -> Gain/1
  Gain/1 -> Product2/1
  Constant/1 -> Product2/2
  Constant1/1 -> Product2/3
  Hr/1 -> Product/1
  Product2/1 -> Product/2
  Product/1 -> eta_fc/1

== system KTH_103002/PEM fuel cell system/Fuel cell stack, Heat Generation/Heat/Heat generation [W] ==
  note: Heat generation [W]
      | --------------------------------
      | Heat=reaheat+ latheat+ sensin-sensout
  sensin : Inport  Port=1  LatchInput=off
  sensout : Inport  Port=2  LatchInput=off
  latheat : Inport  Port=3  LatchInput=off
  reaheat : Inport  Port=4  LatchInput=off
  Display : Display
      settings: Format=short
  Sum : Sum  Inputs=|+-  SaturateOnIntegerOverflow=on
  Sum1 : Sum  Inputs=|++  SaturateOnIntegerOverflow=on
  Sum2 : Sum  Inputs=|++  SaturateOnIntegerOverflow=on
  Heat_fc : Outport  Port=1
  wires:
  sensin/1 -> Sum/1
  sensout/1 -> Sum/2
  Sum/1 -> Sum1/1
  latheat/1 -> Sum1/2
  Sum1/1 -> Sum2/1
  reaheat/1 -> Sum2/2
  Sum2/1 -> Heat_fc/1, Display/1

== system KTH_103002/PEM fuel cell system/Fuel cell stack, Heat Generation/Heat/Latent heat [W] ==
  note: Latent heat
      | ---------------------
      | latheat= Hcond*NWcond
  NWcond : Inport  Port=1  LatchInput=off
  Display : Display
      settings: Format=short
  Heat of condensation : Subsystem
      settings: RTWFcnNameOpts=Auto  RTWFileNameOpts=Auto
  Product : Product  Inputs=2  Multiplication=Element-wise(.*)  SaturateOnIntegerOverflow=on
  latheat [W] : Outport  Port=1
  wires:
  NWcond/1 -> Product/1
  Heat of condensation/1(Hcond [J/mol]) -> Product/2
  Product/1 -> latheat [W]/1, Display/1

== system KTH_103002/PEM fuel cell system/Fuel cell stack, Heat Generation/Heat/Reaction heat [W] ==
  note: Reaction heat [W]
      | -------------------------------
      | NHion = 2*i*A/(2*F);
      | reaheat = (-Hr - 2*F*Ecell)*NHion;
  Current density : Inport  Port=1  LatchInput=off
  Ecell : Inport  Port=2  LatchInput=off
  Constant : Constant  Value=FC.Const.F
  Constant1 : Constant  Value=FC.Const.F
  Constant2 : Constant  Value=FC.Stack.Cell.Dim.A
  Constant3 : Constant  Value=2
  Display : Display
      settings: Format=short
  Gain : Gain  Gain=-1  Multiplication=Element-wise(K.*u)  SaturateOnIntegerOverflow=on
  Heat of reaction : Subsystem
      settings: RTWFcnNameOpts=Auto  RTWFileNameOpts=Auto
  NHion : Product  Inputs=*/  Multiplication=Element-wise(.*)  SaturateOnIntegerOverflow=on
  Product : Product  Inputs=2  Multiplication=Element-wise(.*)  SaturateOnIntegerOverflow=on
  Product1 : Product  Inputs=2  Multiplication=Element-wise(.*)  SaturateOnIntegerOverflow=on
  Product2 : Product  Inputs=3  Multiplication=Element-wise(.*)  SaturateOnIntegerOverflow=on
  Sum : Sum  Inputs=|+-  SaturateOnIntegerOverflow=on
  reaheat [W] : Outport  Port=1
  Hr [J/mol] : Outport  Port=2
  wires:
  Current density/1 -> Product1/1
  Constant2/1 -> Product1/2
  Product1/1 -> NHion/1
  Constant/1 -> NHion/2
  NHion/1 -> Product/1
  Product/1 -> reaheat [W]/1, Display/1
  Heat of reaction/1(Hr [J/mol]) -> Gain/1, Hr [J/mol]/1
  Ecell/1 -> Product2/1
  Constant1/1 -> Product2/2
  Constant3/1 -> Product2/3
  Gain/1 -> Sum/1
  Product2/1 -> Sum/2
  Sum/1 -> Product/2

== system KTH_103002/PEM fuel cell system/Fuel cell stack, Heat Generation/Heat/Sensible heat [W] ==
  note: Sensible heat in and out [W]
      | ------------------------------------------------
      | sensouta = NoutWag*HWgout + NoutHa*HHout+NoutWal*HWl;
      | sensoutc = NoutWcg*HWgout + NoutWcl*HWl + NoutO*HOout + NoutN*HNout;
      |
      | sensin = sensina + sensinc;
      | sensout = sensouta + sensoutc;
  NinWa : Inport  Port=1  LatchInput=off
  NinHa : Inport  Port=2  LatchInput=off
  NoutWag : Inport  Port=3  LatchInput=off
  NoutHa : Inport  Port=4  LatchInput=off
  NinWc : Inport  Port=5  LatchInput=off
  NinO : Inport  Port=6  LatchInput=off
  NInN : Inport  Port=7  LatchInput=off
  NoutWcg : Inport  Port=8  LatchInput=off
  NoutWcl : Inport  Port=9  LatchInput=off
  NoutO : Inport  Port=10  LatchInput=off
  NoutN : Inport  Port=11  LatchInput=off
  Display : Display
      settings: Format=short
  Display1 : Display
      settings: Format=short
  "Sensible heat in " : Subsystem
      settings: RTWFcnNameOpts=Auto  RTWFileNameOpts=Auto
  Sensible heat out : Subsystem
      settings: RTWFcnNameOpts=Auto  RTWFileNameOpts=Auto
  Sum : Sum  Inputs=|++  SaturateOnIntegerOverflow=on
  Sum1 : Sum  Inputs=|++  SaturateOnIntegerOverflow=on
  sensin : Outport  Port=1
  sensout : Outport  Port=2
  wires:
  "Sensible heat in "/1(sensina [W]) -> Sum/1
  NinWa/1 -> "Sensible heat in "/1(NinWa)
  NinHa/1 -> "Sensible heat in "/2(NinHa)
  NinWc/1 -> "Sensible heat in "/3(NinWc)
  NinO/1 -> "Sensible heat in "/4(NinO)
  NInN/1 -> "Sensible heat in "/5(NinN)
  "Sensible heat in "/2(sensinc [W]) -> Sum/2
  NoutWag/1 -> Sensible heat out/1(NoutWag)
  NoutHa/1 -> Sensible heat out/2(NoutHa)
  NoutWcg/1 -> Sensible heat out/3(NoutWcg)
  NoutO/1 -> Sensible heat out/4(NoutO)
  NoutN/1 -> Sensible heat out/5(NoutN)
  NoutWcl/1 -> Sensible heat out/6(NoutWcl)
  Sum/1 -> sensin/1, Display/1
  Sensible heat out/1(sensouta [W]) -> Sum1/1
  Sensible heat out/2(sensoutc [W]) -> Sum1/2
  Sum1/1 -> sensout/1, Display1/1

== system KTH_103002/PEM fuel cell system/Humidifiers/Evapcooler/Ambient air ==
  note: Ambient air
  Humidity in air : Subsystem
      settings: RTWFcnNameOpts=Auto  RTWFileNameOpts=Auto
  Saturation pressure : Subsystem
      settings: RTWFcnNameOpts=Auto  RTWFileNameOpts=Auto
  wires:
  Saturation pressure/1(psat_air) -> Humidity in air/1(psat_air)

== system KTH_103002/PEM fuel cell system/Subsystem1/Anode init/Anode water molar fraction ==
  note: Water molar fraction in the anode inlet stream
  psatah [bar] : Inport  Port=1  LatchInput=off
  Constant1 : Constant  Value=FC.Lab.P.a
  Constant3 : Constant  Value=FC.Lab.Stoich.RHah
  Constant4 : Constant  Value=100
  Product : Product  Inputs=*/  Multiplication=Element-wise(.*)  SaturateOnIntegerOverflow=on
  Product1 : Product  Inputs=*/  Multiplication=Element-wise(.*)  SaturateOnIntegerOverflow=on
  Product2 : Product  Inputs=2  Multiplication=Element-wise(.*)  SaturateOnIntegerOverflow=on
  XWaI [-] : Outport  Port=1
  tag scope: XWaI=global
  wires:
  Constant3/1 -> Product1/1
  Constant4/1 -> Product1/2
  psatah [bar]/1 -> Product/1
  Constant1/1 -> Product/2
  Product1/1 -> Product2/1
  Product/1 -> Product2/2
  Product2/1 -> XWaI [-]/1, [XWaI]
